simulink model "Vorlage_Gesamtanlage_v27"  (R2021a)
settings: Solver=ode3  StartTime=0.0  StopTime=400  FixedStep=0.01  MaxStep=1  MinStep=0.005  RelTol=1e-3  AbsTol=10  EnableMultiTasking=on
undefined symbols (not defined in the file): A, Flaschengroesse, I, igetr, K, Limits, MaxFlaschen, MRK, numA, PassSilo1, PassSilo2, PHI, Ra, SizeSilo1, SizeSilo2, U, v_band_abfuhr_set, v_band_arbeit_set, v_band_zufuhr_set, v_umsetzer_greifer_set, v_umsetzer_set, v_ve1_set, v_ve2_set
libraries: simulink x94
(part 2 of 3)

== system Vorlage_Gesamtanlage_v27/Abfüllanlage/Fehlererkennung/Leere Flasche durch Ve2 ==
  Leere Flasche durch VE2 : Assertion
  Logical Operator1 : Logic  AllPortsSameDT=off  OutDataTypeStr=boolean
  Logical Operator15 : Logic  Operator=NOT  AllPortsSameDT=off  OutDataTypeStr=boolean
  Memory : Memory  InitialCondition=1  InheritSampleTime=on
  Rising Edge : Subsystem
  nac : Outport
  wires:
  Logical Operator15/1 -> Memory/1
  Memory/1 -> Leere Flasche durch VE2/1
  Logical Operator1/1 -> Logical Operator15/1, nac/1
  Rising Edge/1(edge) -> Logical Operator1/2
  [i_dp_ve2_LT_vorne] -> Logical Operator1/1
  [o_dp_ve2] -> Rising Edge/1(signal)

== system Vorlage_Gesamtanlage_v27/Abfüllanlage/Fehlererkennung/Leere Flasche zurueck ==
  Falling Edge : Subsystem
  Leere Flasche zurueck : Assertion
  Logical Operator12 : Logic  Inputs=3  AllPortsSameDT=off  OutDataTypeStr=boolean
  Logical Operator15 : Logic  Operator=NOT  AllPortsSameDT=off  OutDataTypeStr=boolean
  Memory : Memory  InitialCondition=1  InheritSampleTime=on
  nac : Outport
  wires:
  Memory/1 -> Leere Flasche zurueck/1
  Logical Operator12/1 -> nac/1, Logical Operator15/1
  Logical Operator15/1 -> Memory/1
  Falling Edge/1(edge) -> Logical Operator12/3
  [i_dp_umsetz_teller] -> Falling Edge/1(signal)
  [i_dp_teller_behaelter_vorne] -> Logical Operator12/1
  [i_dp_umsetz_greifer_zu] -> Logical Operator12/2

== system Vorlage_Gesamtanlage_v27/Abfüllanlage/Fehlererkennung/Lückenhafte Teller Bestückung ==
  Compare To Zero : simulink/Logic and Bit Operations/Compare To Zero  relop=>  OutDataTypeStr=boolean
  Interval Test : simulink/Logic and Bit Operations/Interval Test  IntervalClosedRight=off  uplimit=405  IntervalClosedLeft=on  lowlimit=0  OutDataTypeStr=boolean
  Logical Operator : Logic  Operator=NOT  AllPortsSameDT=off  OutDataTypeStr=boolean
  Logical Operator1 : Logic  Inputs=3  AllPortsSameDT=off  OutDataTypeStr=boolean
  Logical Operator2 : Logic  Operator=NOT  AllPortsSameDT=off  OutDataTypeStr=boolean
  Lückehafte Tellerbestückung : Assertion
  Memory2 : Memory  InitialCondition=1  InheritSampleTime=on
  Sum of Elements : Sum  Inputs=+
  rising edge : Subsystem
  nac : Outport
  wires:
  Logical Operator2/1 -> Memory2/1
  Memory2/1 -> Lückehafte Tellerbestückung/1
  [Flaschenpositionen] -> Interval Test/1
  Interval Test/1 -> Sum of Elements/1
  Sum of Elements/1 -> Compare To Zero/1
  [o_dp_teller] -> rising edge/1(In1)
  [i_dp_teller_behaelter_vorne] -> Logical Operator/1
  Logical Operator/1 -> Logical Operator1/1  "keine neue Flasche da"
  rising edge/1(Out1) -> Logical Operator1/2  "teller startet"
  Compare To Zero/1 -> Logical Operator1/3  "neue Flaschen vorhanden"
  Logical Operator1/1 -> nac/1, Logical Operator2/1

== system Vorlage_Gesamtanlage_v27/Abfüllanlage/Fehlererkennung/Nachrieseln ==
  Compare To Constant : simulink/Logic and Bit Operations/Compare To Constant  relop===  const=1  OutDataTypeStr=uint8  ZeroCross=off
  Compare To Constant1 : simulink/Logic and Bit Operations/Compare To Constant  relop=<  const=2  OutDataTypeStr=uint8  ZeroCross=off
  Compare To Constant2 : simulink/Logic and Bit Operations/Compare To Constant  relop=>  const=0  OutDataTypeStr=uint8  ZeroCross=off
  Data Type Conversion : DataTypeConversion
  Integrator : Integrator  ExternalReset=rising
  Logical Operator : Logic  Inputs=3  AllPortsSameDT=off  OutDataTypeStr=boolean
  Logical Operator1 : Logic  Operator=NOT  AllPortsSameDT=off  OutDataTypeStr=boolean
  Logical Operator3 : Logic  Operator=NOT  AllPortsSameDT=off  OutDataTypeStr=boolean
  Memory2 : Memory  InitialCondition=1  InheritSampleTime=on
  Nachrieselzeit missachtet : Assertion
  Rising Edge1 : Subsystem
  nac : Outport
  wires:
  Rising Edge1/1(edge) -> Compare To Constant/1
  Compare To Constant/1 -> Logical Operator/3
  Compare To Constant1/1 -> Logical Operator/2
  Integrator/1 -> Compare To Constant1/1, Compare To Constant2/1
  Logical Operator/1 -> nac/1, Logical Operator3/1
  Logical Operator3/1 -> Memory2/1
  Memory2/1 -> Nachrieselzeit missachtet/1
  [i_dp_BEKenn_LS_oben] -> Logical Operator1/1
  Logical Operator1/1 -> Data Type Conversion/1
  [o_dp_teller] -> Rising Edge1/1(signal)
  Data Type Conversion/1 -> Integrator/1, Integrator/2
  Compare To Constant2/1 -> Logical Operator/1

== system Vorlage_Gesamtanlage_v27/Abfüllanlage/Fehlererkennung/Sinnloser Schaltvorgang Ve1 ==
  CompareTo Constant12 : simulink/Logic and Bit Operations/Compare To Constant  relop===  const=0  OutDataTypeStr=boolean  ZeroCross=off
  Logical Operator1 : Logic  AllPortsSameDT=off  OutDataTypeStr=boolean
  Logical Operator17 : Logic  Operator=NOT  AllPortsSameDT=off  OutDataTypeStr=boolean
  Memory1 : Memory  InitialCondition=1  InheritSampleTime=on
  Rising Edge : Subsystem
  Sinnloser Schaltvorgang VE1 : Assertion
  nac : Outport
  wires:
  [o_dp_ve1] -> Rising Edge/1(signal)
  [i_dp_ve1_LT] -> CompareTo Constant12/1
  Logical Operator1/1 -> nac/1, Logical Operator17/1
  CompareTo Constant12/1 -> Logical Operator1/1
  Rising Edge/1(edge) -> Logical Operator1/2
  Memory1/1 -> Sinnloser Schaltvorgang VE1/1
  Logical Operator17/1 -> Memory1/1

== system Vorlage_Gesamtanlage_v27/Abfüllanlage/Fehlererkennung/Sinnloser Schaltvorgang Ve2 ==
  CompareTo Constant12 : simulink/Logic and Bit Operations/Compare To Constant  relop===  const=0  OutDataTypeStr=boolean  ZeroCross=off
  Logical Operator1 : Logic  AllPortsSameDT=off  OutDataTypeStr=boolean
  Logical Operator17 : Logic  Operator=NOT  AllPortsSameDT=off  OutDataTypeStr=boolean
  Memory1 : Memory  InitialCondition=1  InheritSampleTime=on
  Rising Edge : Subsystem
  Sinnloser Schaltvorgang VE2 : Assertion
  nac2 : Outport
  wires:
  Logical Operator17/1 -> Memory1/1
  Memory1/1 -> Sinnloser Schaltvorgang VE2/1
  Rising Edge/1(edge) -> Logical Operator1/2
  CompareTo Constant12/1 -> Logical Operator1/1
  Logical Operator1/1 -> Logical Operator17/1, nac2/1
  [i_dp_ve2_LT] -> CompareTo Constant12/1
  [o_dp_ve2] -> Rising Edge/1(signal)

== system Vorlage_Gesamtanlage_v27/Abfüllanlage/Fehlererkennung/Teller dreht obwohl Flasche nicht gefuellt ==
  CompareTo Constant11 : simulink/Logic and Bit Operations/Compare To Constant  relop===  const=1  OutDataTypeStr=boolean  ZeroCross=off
  CompareTo Constant12 : simulink/Logic and Bit Operations/Compare To Constant  relop===  const=1  OutDataTypeStr=boolean  ZeroCross=off
  Logical Operator15 : Logic  Operator=NOT  AllPortsSameDT=off  OutDataTypeStr=boolean
  Logical Operator17 : Logic  Inputs=3  AllPortsSameDT=off  OutDataTypeStr=boolean
  Memory : Memory  InitialCondition=1  InheritSampleTime=on
  Rising Edge : Subsystem
  Teller dreht obwohl Flasche nicht gefüllt : Assertion
  nac : Outport
  wires:
  Logical Operator15/1 -> Memory/1
  Memory/1 -> Teller dreht obwohl Flasche nicht gefüllt/1
  CompareTo Constant11/1 -> Logical Operator17/1
  CompareTo Constant12/1 -> Logical Operator17/2
  Rising Edge/1(edge) -> Logical Operator17/3
  Logical Operator17/1 -> Logical Operator15/1, nac/1
  [i_dp_BEKenn_LS_oben] -> CompareTo Constant11/1
  [i_dp_BEKenn_LT_unten] -> CompareTo Constant12/1
  [o_dp_teller] -> Rising Edge/1(signal)

== system Vorlage_Gesamtanlage_v27/Abfüllanlage/Fehlererkennung/Teller dreht obwohl Greifer zu ==
  note: Changelog v23 -> v24:
      | o_dp_umsetz_teller geändert zu i_dp_umsetz_teller
      | o_dp_umsetz_greifer_zu geändert zu i_dp_umsetz_greifer_zu
  Logical Operator14 : Logic  Inputs=4  AllPortsSameDT=off  OutDataTypeStr=boolean
  Logical Operator15 : Logic  Operator=NOT  AllPortsSameDT=off  OutDataTypeStr=boolean
  Memory12 : Memory  InitialCondition=1
  Teller dreht obwohl Greifer zu : Assertion
  nac : Outport
  wires:
  Logical Operator15/1 -> Memory12/1
  Memory12/1 -> Teller dreht obwohl Greifer zu/1
  Logical Operator14/1 -> Logical Operator15/1, nac/1
  [i_dp_umsetz_teller] -> Logical Operator14/1
  [i_dp_umsetz_greifer_zu] -> Logical Operator14/2
  [i_dp_teller_behaelter] -> Logical Operator14/3
  [o_dp_teller] -> Logical Operator14/4

== system Vorlage_Gesamtanlage_v27/Abfüllanlage/Fehlererkennung/Teller dreht volle Flasche durch ==
  Logical Operator1 : Logic  Operator=NOT  AllPortsSameDT=off  OutDataTypeStr=boolean
  Logical Operator2 : Logic  AllPortsSameDT=off  OutDataTypeStr=boolean
  Memory1 : Memory  InitialCondition=1  InheritSampleTime=on
  Rising Edge : Subsystem
  Teller dreht volle Flasche durch : Assertion
  nac1 : Outport
  wires:
  Memory1/1 -> Teller dreht volle Flasche durch/1
  Logical Operator1/1 -> Memory1/1
  Logical Operator2/1 -> Logical Operator1/1, nac1/1
  Rising Edge/1(edge) -> Logical Operator2/2
  [o_dp_teller] -> Rising Edge/1(signal)
  [i_dp_teller_behaelter_hinten] -> Logical Operator2/1

== system Vorlage_Gesamtanlage_v27/Abfüllanlage/Fehlererkennung/Triggered Subsystem13 ==
  Flaschenpositionen : Inport
  CompareTo Constant11 : simulink/Logic and Bit Operations/Compare To Constant  relop=>  const=0  OutDataTypeStr=boolean  ZeroCross=off
  Interval Test10 : simulink/Logic and Bit Operations/Interval Test  IntervalClosedRight=off  uplimit=405.2  IntervalClosedLeft=off  lowlimit=404.8  OutDataTypeStr=boolean
  Sum of Elements9 : Sum  Inputs=+
  i_dp_teller_behaelter_vorne : Outport
  wires:
  Flaschenpositionen/1 -> Interval Test10/1
  Interval Test10/1 -> Sum of Elements9/1
  Sum of Elements9/1 -> CompareTo Constant11/1
  CompareTo Constant11/1 -> i_dp_teller_behaelter_vorne/1

== system Vorlage_Gesamtanlage_v27/Abfüllanlage/Fehlererkennung/Triggered Subsystem14 ==
  Flaschenpositionen : Inport
  CompareTo Constant11 : simulink/Logic and Bit Operations/Compare To Constant  relop=>  const=0  OutDataTypeStr=boolean  ZeroCross=off
  Interval Test10 : simulink/Logic and Bit Operations/Interval Test  IntervalClosedRight=off  uplimit=305.2  IntervalClosedLeft=off  lowlimit=304.8  OutDataTypeStr=boolean
  Sum of Elements9 : Sum  Inputs=+
  i_dp_ve2_LT_vorne : Outport
  wires:
  Flaschenpositionen/1 -> Interval Test10/1
  Interval Test10/1 -> Sum of Elements9/1
  Sum of Elements9/1 -> CompareTo Constant11/1
  CompareTo Constant11/1 -> i_dp_ve2_LT_vorne/1

== system Vorlage_Gesamtanlage_v27/Abfüllanlage/Fehlererkennung/Triggered Subsystem15 ==
  Flaschenpositionen : Inport
  CompareTo Constant11 : simulink/Logic and Bit Operations/Compare To Constant  relop=>  const=0  OutDataTypeStr=boolean  ZeroCross=off
  Interval Test10 : simulink/Logic and Bit Operations/Interval Test  IntervalClosedRight=off  uplimit=505.2  IntervalClosedLeft=off  lowlimit=504.8  OutDataTypeStr=boolean
  Sum of Elements9 : Sum  Inputs=+
  i_dp_teller_behaelter_hinten : Outport
  wires:
  CompareTo Constant11/1 -> i_dp_teller_behaelter_hinten/1
  Sum of Elements9/1 -> CompareTo Constant11/1
  Interval Test10/1 -> Sum of Elements9/1
  Flaschenpositionen/1 -> Interval Test10/1

== system Vorlage_Gesamtanlage_v27/Abfüllanlage/Fehlererkennung/Triggered Subsystem16 ==
  Flaschenpositionen : Inport
  CompareTo Constant11 : simulink/Logic and Bit Operations/Compare To Constant  relop=>  const=0  OutDataTypeStr=boolean  ZeroCross=off
  Interval Test10 : simulink/Logic and Bit Operations/Interval Test  IntervalClosedRight=off  uplimit=605.2  IntervalClosedLeft=off  lowlimit=604.8  OutDataTypeStr=boolean
  Sum of Elements9 : Sum  Inputs=+
  i_dp_ve2_LT_hinten : Outport
  wires:
  Flaschenpositionen/1 -> Interval Test10/1
  Interval Test10/1 -> Sum of Elements9/1
  Sum of Elements9/1 -> CompareTo Constant11/1
  CompareTo Constant11/1 -> i_dp_ve2_LT_hinten/1

== system Vorlage_Gesamtanlage_v27/Abfüllanlage/Fehlererkennung/Umsetzerpneumatik beschädigt ==
  Logical Operator23 : Logic  Operator=NOT  AllPortsSameDT=off  OutDataTypeStr=boolean
  Logical Operator24 : Logic  AllPortsSameDT=off  OutDataTypeStr=boolean
  Memory9 : Memory  InitialCondition=1
  Umsetzerpneumatik beschädigt : Assertion
  nac : Outport
  wires:
  Logical Operator24/1 -> Logical Operator23/1, nac/1
  Logical Operator23/1 -> Memory9/1
  Memory9/1 -> Umsetzerpneumatik beschädigt/1
  [o_dp_umsetz_band] -> Logical Operator24/1
  [o_dp_umsetz_teller] -> Logical Operator24/2

== system Vorlage_Gesamtanlage_v27/Abfüllanlage/Fehlererkennung/Vereinzeler1 schließt mit Flasche ==
  Compare To Constant : simulink/Logic and Bit Operations/Compare To Constant  relop=>=  const=1  OutDataTypeStr=boolean
  Interval Test : simulink/Logic and Bit Operations/Interval Test  IntervalClosedRight=off  uplimit=205  IntervalClosedLeft=off  lowlimit=201  OutDataTypeStr=boolean
  Logical Operator : Logic  AllPortsSameDT=off  OutDataTypeStr=boolean
  Logical Operator2 : Logic  Operator=NOT  AllPortsSameDT=off  OutDataTypeStr=boolean
  Memory2 : Memory  InitialCondition=1  InheritSampleTime=on
  Sum of Elements : Sum  Inputs=+
  Vereinzeler1 schließt mit Flasche : Assertion
  falling edge : Subsystem
  nac : Outport
  wires:
  Memory2/1 -> Vereinzeler1 schließt mit Flasche/1
  Logical Operator2/1 -> Memory2/1
  [o_dp_ve1] -> falling edge/1(In1)
  [Flaschenpositionen] -> Interval Test/1
  Interval Test/1 -> Sum of Elements/1
  Sum of Elements/1 -> Compare To Constant/1
  falling edge/1(Out1) -> Logical Operator/1
  Compare To Constant/1 -> Logical Operator/2
  Logical Operator/1 -> nac/1, Logical Operator2/1

== system Vorlage_Gesamtanlage_v27/Abfüllanlage/Fehlererkennung/Vereinzeler2 schließt mit Flasche1 ==
  Compare To Constant : simulink/Logic and Bit Operations/Compare To Constant  relop=>=  const=1  OutDataTypeStr=boolean
  Interval Test : simulink/Logic and Bit Operations/Interval Test  IntervalClosedRight=off  uplimit=610  IntervalClosedLeft=on  lowlimit=605  OutDataTypeStr=boolean
  Logical Operator : Logic  AllPortsSameDT=off  OutDataTypeStr=boolean
  Logical Operator2 : Logic  Operator=NOT  AllPortsSameDT=off  OutDataTypeStr=boolean
  Memory2 : Memory  InitialCondition=1  InheritSampleTime=on
  Sum of Elements : Sum  Inputs=+
  Vereinzeler2 schließt mit Flasche : Assertion
  falling edge : Subsystem
  nac : Outport
  wires:
  Logical Operator/1 -> nac/1, Logical Operator2/1
  Compare To Constant/1 -> Logical Operator/2
  falling edge/1(Out1) -> Logical Operator/1
  Sum of Elements/1 -> Compare To Constant/1
  Interval Test/1 -> Sum of Elements/1
  [Flaschenpositionen] -> Interval Test/1
  [o_dp_ve2] -> falling edge/1(In1)
  Logical Operator2/1 -> Memory2/1
  Memory2/1 -> Vereinzeler2 schließt mit Flasche/1

== system Vorlage_Gesamtanlage_v27/Abfüllanlage/Fehlererkennung/Volle Flasche zum Teller zurück ==
  Chart : Stateflow chart  TreatAsAtomicUnit=on
  Logical Operator2 : Logic  Operator=NOT  AllPortsSameDT=off  OutDataTypeStr=boolean
  Memory2 : Memory  InitialCondition=1  InheritSampleTime=on
  Scope : Scope
  Volle Flasche zum Teller zurueck : Assertion
  nac : Outport
  wires:
  Logical Operator2/1 -> Memory2/1
  Memory2/1 -> Volle Flasche zum Teller zurueck/1
  Chart/1(error) -> nac/1, Logical Operator2/1
  [i_dp_ve2_herein] -> Scope/1, Chart/6(i_ve2_herein)
  [i_dp_umsetz_band] -> Chart/5(i_umsetz_band)
  [i_dp_umsetz_greifer_auf] -> Chart/4(i_greifer_auf)
  [i_dp_umsetz_teller] -> Chart/3(i_umsetz_teller)
  [i_dp_teller_behaelter_hinten] -> Chart/1(I_teller_behaelter_hinten)
  [i_dp_umsetz_greifer_zu] -> Chart/2(i_greifer_zu)
  [o_dp_umsetz_teller] -> Chart/7(o_umsetz_teller)

== system Vorlage_Gesamtanlage_v27/Abfüllanlage/Fehlererkennung/Volle Flasche zurueck ==
  Falling Edge : Subsystem
  Logical Operator1 : Logic  Inputs=3  AllPortsSameDT=off  OutDataTypeStr=boolean
  Logical Operator15 : Logic  Operator=NOT  AllPortsSameDT=off  OutDataTypeStr=boolean
  Memory : Memory  InitialCondition=1  InheritSampleTime=on
  Volle Flasche zurueck : Assertion
  nac : Outport
  wires:
  Logical Operator15/1 -> Memory/1
  Logical Operator1/1 -> Logical Operator15/1, nac/1
  Memory/1 -> Volle Flasche zurueck/1
  Falling Edge/1(edge) -> Logical Operator1/3
  [i_dp_umsetz_band] -> Falling Edge/1(signal)
  [i_dp_ve2_LT_hinten] -> Logical Operator1/1
  [i_dp_umsetz_greifer_zu] -> Logical Operator1/2

== system Vorlage_Gesamtanlage_v27/Abfüllanlage/Fehlererkennung/Zwei Flaschen im Umsetzer1 ==
  CompareTo Constant2 : simulink/Logic and Bit Operations/Compare To Constant  relop=>  const=1  OutDataTypeStr=boolean  ZeroCross=off
  Interval Test2 : simulink/Logic and Bit Operations/Interval Test  IntervalClosedRight=off  uplimit=405  IntervalClosedLeft=on  lowlimit=306  OutDataTypeStr=boolean
  Logical Operator2 : Logic  Operator=NOT  AllPortsSameDT=off  OutDataTypeStr=boolean
  Memory4 : Memory  InitialCondition=1
  Sum of Elements2 : Sum  Inputs=+
  Zwei Flaschen im Umsetzer1 : Assertion
  nac : Outport
  wires:
  Sum of Elements2/1 -> CompareTo Constant2/1
  Interval Test2/1 -> Sum of Elements2/1
  Logical Operator2/1 -> Memory4/1
  CompareTo Constant2/1 -> Logical Operator2/1, nac/1
  Memory4/1 -> Zwei Flaschen im Umsetzer1/1
  [Flaschenpositionen] -> Interval Test2/1

== system Vorlage_Gesamtanlage_v27/Abfüllanlage/Fehlererkennung/Zwei Flaschen im Umsetzer2 ==
  CompareTo Constant3 : simulink/Logic and Bit Operations/Compare To Constant  relop=>  const=1  OutDataTypeStr=boolean  ZeroCross=off
  Interval Test3 : simulink/Logic and Bit Operations/Interval Test  IntervalClosedRight=off  uplimit=604  IntervalClosedLeft=on  lowlimit=505  OutDataTypeStr=boolean
  Logical Operator3 : Logic  Operator=NOT  AllPortsSameDT=off  OutDataTypeStr=boolean
  Memory3 : Memory  InitialCondition=1
  Sum of Elements3 : Sum  Inputs=+
  Zwei Flaschen im Umsetzer2 : Assertion
  nac : Outport
  wires:
  Sum of Elements3/1 -> CompareTo Constant3/1
  Interval Test3/1 -> Sum of Elements3/1
  Logical Operator3/1 -> Memory3/1
  CompareTo Constant3/1 -> Logical Operator3/1, nac/1
  Memory3/1 -> Zwei Flaschen im Umsetzer2/1
  [Flaschenpositionen] -> Interval Test3/1

== system Vorlage_Gesamtanlage_v27/Abfüllanlage/Fehlererkennung/Zwei Flaschen im Ve1 ==
  CompareTo Constant : simulink/Logic and Bit Operations/Compare To Constant  relop=>  const=1  OutDataTypeStr=boolean  ZeroCross=off
  Interval Test : simulink/Logic and Bit Operations/Interval Test  IntervalClosedRight=off  uplimit=205  IntervalClosedLeft=on  lowlimit=201  OutDataTypeStr=boolean
  Logical Operator : Logic  Operator=NOT  AllPortsSameDT=off  OutDataTypeStr=boolean
  Memory6 : Memory  InitialCondition=1
  Sum of Elements : Sum  Inputs=+
  Zwei Flaschen im Ve1 : Assertion
  nac : Outport
  wires:
  Memory6/1 -> Zwei Flaschen im Ve1/1
  CompareTo Constant/1 -> Logical Operator/1, nac/1
  Logical Operator/1 -> Memory6/1
  Interval Test/1 -> Sum of Elements/1
  Sum of Elements/1 -> CompareTo Constant/1
  [Flaschenpositionen] -> Interval Test/1

== system Vorlage_Gesamtanlage_v27/Abfüllanlage/Fehlererkennung/Zwei Flaschen im Ve2 ==
  CompareTo Constant1 : simulink/Logic and Bit Operations/Compare To Constant  relop=>  const=1  OutDataTypeStr=boolean  ZeroCross=off
  Interval Test1 : simulink/Logic and Bit Operations/Interval Test  IntervalClosedRight=off  uplimit=610  IntervalClosedLeft=on  lowlimit=605  OutDataTypeStr=boolean
  Interval Test2 : simulink/Logic and Bit Operations/Interval Test  IntervalClosedRight=off  uplimit=305  IntervalClosedLeft=on  lowlimit=300  OutDataTypeStr=boolean
  Logical Operator : Logic  Operator=OR  AllPortsSameDT=off  OutDataTypeStr=boolean
  Logical Operator1 : Logic  Operator=NOT  AllPortsSameDT=off  OutDataTypeStr=boolean
  Memory5 : Memory  InitialCondition=1
  Sum of Elements1 : Sum  Inputs=+
  Zwei Flaschen im Ve2 : Assertion
  nac : Outport
  wires:
  Sum of Elements1/1 -> CompareTo Constant1/1
  Logical Operator1/1 -> Memory5/1
  CompareTo Constant1/1 -> Logical Operator1/1, nac/1
  Memory5/1 -> Zwei Flaschen im Ve2/1
  [Flaschenpositionen] -> Interval Test1/1, Interval Test2/1
  Interval Test1/1 -> Logical Operator/1
  Interval Test2/1 -> Logical Operator/2
  Logical Operator/1 -> Sum of Elements1/1

== system Vorlage_Gesamtanlage_v27/Abfüllanlage/Fehlererkennung/nac ==
  nac : Inport
  Constant : Constant  Value=numA
  Data Type Conversion2 : DataTypeConversion  OutDataTypeStr=double
  Display : Display
  Increment Stored Integer : simulink/Additional Math & Discrete/Additional Math: Increment - Decrement/Increment Stored Integer
  MinMax : MinMax  Function=max  Inputs=2
  Product1 : Product  RndMeth=Zero
  To Workspace : ToWorkspace  VariableName=numA  SampleTime=-1
      settings: MaxDataPoints=1
  wires:
  nac/1 -> Data Type Conversion2/1
  MinMax/1 -> Display/1, To Workspace/1
  Constant/1 -> Increment Stored Integer/1, MinMax/1
  Increment Stored Integer/1 -> Product1/1
  Data Type Conversion2/1 -> Product1/2
  Product1/1 -> MinMax/2

== system Vorlage_Gesamtanlage_v27/Abfüllanlage/Flaschen_data/Flaschengeschwindigkeiten ==
  Anlagengeschwindigkeiten : Inport
  i_dp_umsetz_greifer_zu : Inport  Port=2
  Flaschenpositionen : Inport  Port=3
  umsetz_pos : Inport  Port=4
  Anlagenpositionsbestimmung : Subsystem
  Filter : Subsystem
  Flaschenabstandsüberwachung : Subsystem
  Product : Product  RndMeth=Zero  SaturateOnIntegerOverflow=on  OutDataTypeStr=Inherit: Same as first input
  Selector : Selector  InputPortWidth=10  IndexOptions=Index vector (port)  Indices=[1 3]  OutputSizes=1
  Flaschengeschwindigkeiten : Outport
  Anlagenpositionen : Outport  Port=2
  tag scope: Anlagenposition=global, Flaschenanlagengeschwindigkeiten=global
  wires:
  Flaschenpositionen/1 -> Anlagenpositionsbestimmung/1(Flaschenposition), Flaschenabstandsüberwachung/1(Flaschenpostionen)
  Anlagenpositionsbestimmung/1(Anlagenposition) -> Selector/2, [Anlagenposition], Anlagenpositionen/1
  Anlagengeschwindigkeiten/1 -> Filter/1(Anlagengeschwindigkeiten)
  Filter/1(Flaschenanlagengeschwindigkeiten) -> Selector/1, [Flaschenanlagengeschwindigkeiten]
  i_dp_umsetz_greifer_zu/1 -> Filter/2(i_dp_umsetz_greifer_zu)
  Flaschenabstandsüberwachung/1(Bewegung möglich) -> Product/2
  Selector/1 -> Product/1
  Product/1 -> Flaschengeschwindigkeiten/1
  umsetz_pos/1 -> Flaschenabstandsüberwachung/2(umsetz_pos)

== system Vorlage_Gesamtanlage_v27/Abfüllanlage/Flaschen_data/Flaschenstarter ==
  Flaschenpositionen : Inport
  Flasche : Inport  Port=2
  Constant : Constant  OutDataTypeStr=uint16
  Flaschenstarter : Subsystem
  Math Function : Math  Operator=mod  SignedPower=on  SaturateOnIntegerOverflow=on
  Maximale Flaschenanzahl : Constant  Value=MaxFlaschen  OutDataTypeStr=uint16
  Memory : Memory  InitialCondition=1
  Sum1 : Sum  Inputs=|++  SaturateOnIntegerOverflow=on
  in_Flaschenzähler : Subsystem
  Flaschenpositionen mit Starter : Outport
  tag scope: Flaschenanzahl=global
  wires:
  in_Flaschenzähler/2(Count) -> Math Function/1
  Maximale Flaschenanzahl/1 -> Math Function/2
  Math Function/1 -> [Flaschenanzahl], Sum1/1
  in_Flaschenzähler/1(Rising Edge) -> Flaschenstarter/3(Rising_edge von Flasche)
  Sum1/1 -> Memory/1
  Constant/1 -> Sum1/2
  Memory/1 -> Flaschenstarter/2(Flaschenanzahl)
  Flaschenpositionen/1 -> Flaschenstarter/1(Flaschenpositionen)
  Flaschenstarter/1(Flaschenpositionen mit Starter) -> Flaschenpositionen mit Starter/1
  Flasche/1 -> in_Flaschenzähler/1(Signal)

== system Vorlage_Gesamtanlage_v27/Abfüllanlage/Flaschen_data/v -> x ==
  Flaschengeschwindigkeiten : Inport
  Anlagenpositionen : Inport  Port=2
  Anlagenlimits : Inport  Port=3
  Compare To Zero : simulink/Logic and Bit Operations/Compare To Zero  relop=>  OutDataTypeStr=boolean  ZeroCross=off
  Data Type Conversion : DataTypeConversion
  Derivative : Derivative
  Gain : Gain  Gain=0
  Integrator : Integrator  ExternalReset=rising  InitialConditionSource=external  InitialCondition=zeros(25,1)  UpperSaturationLimit=Limits  LowerSaturationLimit=[0 0 0]
  Memory : Memory  InitialCondition=ones(25,1)*100
  Memory1 : Memory  InitialCondition=ones(25,1)
  Saturation Dynamic : simulink/Discontinuities/Saturation Dynamic  OutMin=[]  OutMax=[]  OutDataTypeStr=Inherit: Same as second input  OutDataType=sfix(16)  OutScaling=2^-10  DoSatur=off
  Selector : Selector  InputPortWidth=10  IndexOptions=Index vector (port)  Indices=[1 3]  OutputSizes=1
  Flaschenpositionen : Outport
  wires:
  Flaschengeschwindigkeiten/1 -> Integrator/1
  Gain/1 -> Saturation Dynamic/3
  Derivative/1 -> Compare To Zero/1
  Compare To Zero/1 -> Data Type Conversion/1
  Anlagenlimits/1 -> Selector/1
  Integrator/1 -> Saturation Dynamic/2
  Saturation Dynamic/1 -> Flaschenpositionen/1
  Anlagenpositionen/1 -> Memory1/1
  Selector/1 -> Derivative/1, Gain/1, Saturation Dynamic/1, Memory/1
  Memory1/1 -> Selector/2
  Memory/1 -> Integrator/3
  Data Type Conversion/1 -> Integrator/2

== system Vorlage_Gesamtanlage_v27/Abfüllanlage/Umsetzgreifer/Greifer ==
  o_dp_umsetz_greifer_auf : Inport
  o_dp_umsetz_greifer_zu : Inport  Port=2
  Compare To Constant2 : simulink/Logic and Bit Operations/Compare To Constant  relop=>=  const=100  OutDataTypeStr=boolean  ZeroCross=off
  Compare To Constant3 : simulink/Logic and Bit Operations/Compare To Constant  relop=<=  const=0  OutDataTypeStr=boolean  ZeroCross=off
  Derivative : Derivative
  Gain2 : Gain  Gain=v_umsetzer_greifer_set
  Integrator1 : Integrator  LimitOutput=on  UpperSaturationLimit=100  LowerSaturationLimit=0
  Subtract1 : Sum  Inputs=+-
  i_dp_umsetz_greifer_auf : Outport  OutDataTypeStr=boolean
  i_dp_umsetz_greifer_zu : Outport  Port=2  OutDataTypeStr=boolean
  tag scope: i_dp_umsetz_greifer_auf=global, i_dp_umsetz_greifer_zu=global, o_dp_umsetz_greifer_auf=global, o_dp_umsetz_greifer_zu=global, s_Greifer=global, v_Greifer=global
  wires:
  Gain2/1 -> Integrator1/1
  Subtract1/1 -> Gain2/1
  Integrator1/1 -> Compare To Constant3/1, [s_Greifer], Compare To Constant2/1, Derivative/1
  o_dp_umsetz_greifer_zu/1 -> Subtract1/2, [o_dp_umsetz_greifer_zu]
  o_dp_umsetz_greifer_auf/1 -> Subtract1/1, [o_dp_umsetz_greifer_auf]
  Compare To Constant2/1 -> i_dp_umsetz_greifer_auf/1, [i_dp_umsetz_greifer_auf]
  Compare To Constant3/1 -> i_dp_umsetz_greifer_zu/1, [i_dp_umsetz_greifer_zu]
  Derivative/1 -> [v_Greifer]

== system Vorlage_Gesamtanlage_v27/Abfüllanlage/Umsetzgreifer/Umsetzer ==
  o_dp_umsetz_band : Inport
  o_dp_umsetz_teller : Inport  Port=2
  Compare To Constant : simulink/Logic and Bit Operations/Compare To Constant  relop=>=  const=100  OutDataTypeStr=boolean  ZeroCross=off
  Compare To Constant1 : simulink/Logic and Bit Operations/Compare To Constant  relop=<=  const=0  OutDataTypeStr=boolean  ZeroCross=off
  Derivative : Derivative
  Gain : Gain  Gain=-v_umsetzer_set
  Integrator : Integrator  InitialCondition=100  LimitOutput=on  UpperSaturationLimit=101  LowerSaturationLimit=0
  Subtract : Sum  Inputs=+-
  v_umsetzer : Outport  OutDataTypeStr=double
  i_dp_umsetz_teller : Outport  Port=2  OutDataTypeStr=boolean
  i_dp_umsetz_band : Outport  Port=3  OutDataTypeStr=boolean
  umsetz_pos : Outport  Port=4  OutDataTypeStr=double
  tag scope: i_dp_umsetz_band=global, i_dp_umsetz_teller=global, o_dp_umsetz_band=global, o_dp_umsetz_teller=global, s_umsetzer=global, v_umsetzer=global
  wires:
  Gain/1 -> Integrator/1
  Subtract/1 -> Gain/1
  Integrator/1 -> Compare To Constant/1, Derivative/1, Compare To Constant1/1, [s_umsetzer], umsetz_pos/1
  o_dp_umsetz_band/1 -> Subtract/1, [o_dp_umsetz_band]
  o_dp_umsetz_teller/1 -> Subtract/2, [o_dp_umsetz_teller]
  Derivative/1 -> v_umsetzer/1, [v_umsetzer]
  Compare To Constant/1 -> i_dp_umsetz_teller/1, [i_dp_umsetz_teller]
  Compare To Constant1/1 -> i_dp_umsetz_band/1, [i_dp_umsetz_band]

== system Vorlage_Gesamtanlage_v27/Auswertung/Gesamt/Flaschenpositionen ==
  Flaschenpositionen : Scope
  To Workspace : ToWorkspace  VariableName=Flaschenpositionen  SaveFormat=Structure With Time  SampleTime=-1
  wires:
  [Flaschenpositionen] -> Flaschenpositionen/1, To Workspace/1  "Flaschenpositionen"

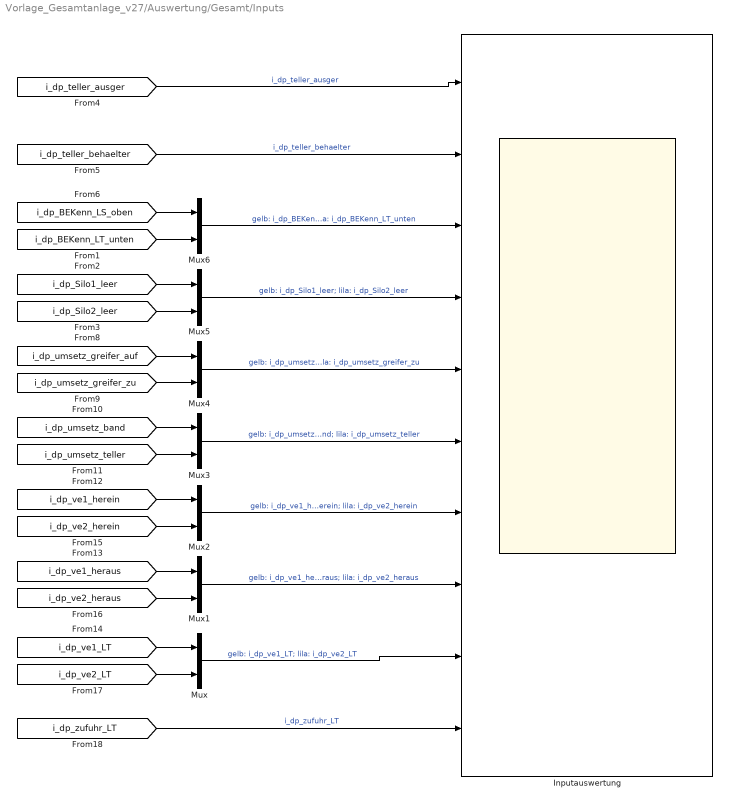
== system Vorlage_Gesamtanlage_v27/Auswertung/Gesamt/Inputs ==
  Inputauswertung : Scope  NumInputPorts=10
  Mux{,1..6} (7 alike) : Mux  Inputs=2
  wires:
  [i_dp_ve1_LT] -> Mux/1
  [i_dp_ve2_LT] -> Mux/2
  [i_dp_ve1_heraus] -> Mux1/1
  [i_dp_ve2_heraus] -> Mux1/2
  [i_dp_ve1_herein] -> Mux2/1
  [i_dp_ve2_herein] -> Mux2/2
  [i_dp_umsetz_band] -> Mux3/1
  [i_dp_umsetz_teller] -> Mux3/2
  [i_dp_umsetz_greifer_auf] -> Mux4/1
  [i_dp_umsetz_greifer_zu] -> Mux4/2
  [i_dp_Silo1_leer] -> Mux5/1
  [i_dp_Silo2_leer] -> Mux5/2
  [i_dp_BEKenn_LS_oben] -> Mux6/1
  [i_dp_BEKenn_LT_unten] -> Mux6/2
  [i_dp_teller_ausger] -> Inputauswertung/1  "i_dp_teller_ausger"
  [i_dp_teller_behaelter] -> Inputauswertung/2  "i_dp_teller_behaelter"
  Mux6/1 -> Inputauswertung/3  "gelb: i_dp_BEKenn_LS_oben; lila: i_dp_BEKenn_LT_unten"
  Mux5/1 -> Inputauswertung/4  "gelb: i_dp_Silo1_leer; lila: i_dp_Silo2_leer"
  Mux4/1 -> Inputauswertung/5  "gelb: i_dp_umsetz_greifer_auf; lila: i_dp_umsetz_greifer_zu"
  Mux3/1 -> Inputauswertung/6  "gelb: i_dp_umsetz_band; lila: i_dp_umsetz_teller"
  Mux2/1 -> Inputauswertung/7  "gelb: i_dp_ve1_herein; lila: i_dp_ve2_herein"
  Mux1/1 -> Inputauswertung/8  "gelb: i_dp_ve1_heraus; lila: i_dp_ve2_heraus"
  [i_dp_zufuhr_LT] -> Inputauswertung/10  "i_dp_zufuhr_LT"
  Mux/1 -> Inputauswertung/9  "gelb: i_dp_ve1_LT; lila: i_dp_ve2_LT"

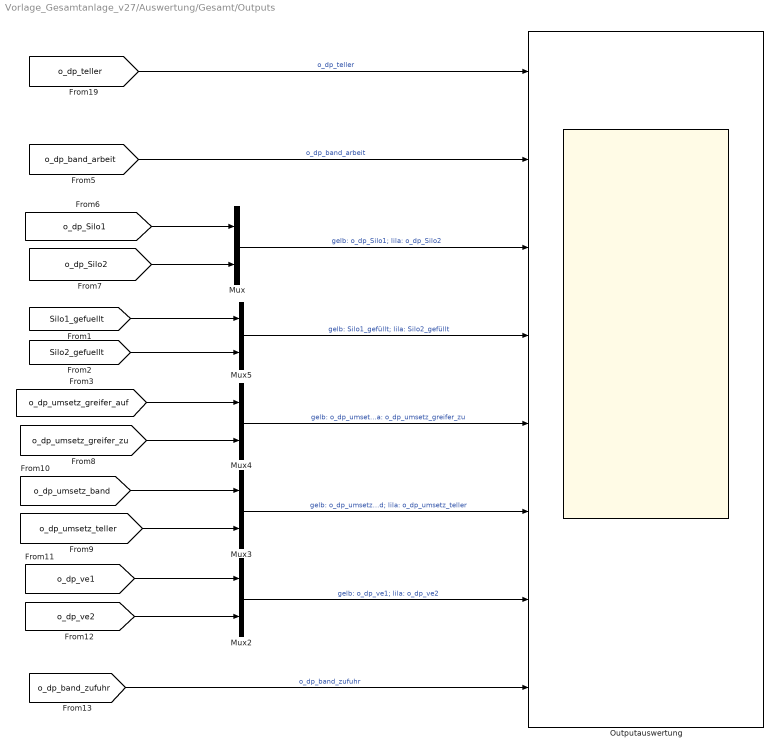
== system Vorlage_Gesamtanlage_v27/Auswertung/Gesamt/Outputs ==
  Mux{,2..5} (5 alike) : Mux  Inputs=2
  Outputauswertung : Scope  NumInputPorts=8
  wires:
  Mux2/1 -> Outputauswertung/7  "gelb: o_dp_ve1; lila: o_dp_ve2"
  Mux3/1 -> Outputauswertung/6  "gelb: o_dp_umsetz_band; lila: o_dp_umsetz_teller"
  Mux4/1 -> Outputauswertung/5  "gelb: o_dp_umsetz_greifer_auf; lila: o_dp_umsetz_greifer_zu"
  Mux5/1 -> Outputauswertung/4  "gelb: Silo1_gefüllt; lila: Silo2_gefüllt"
  [o_dp_band_arbeit] -> Outputauswertung/2  "o_dp_band_arbeit"
  [o_dp_teller] -> Outputauswertung/1  "o_dp_teller"
  [o_dp_umsetz_greifer_zu] -> Mux4/2
  [o_dp_umsetz_greifer_auf] -> Mux4/1
  [o_dp_umsetz_band] -> Mux3/1
  [o_dp_umsetz_teller] -> Mux3/2
  [Silo2_gefuellt] -> Mux5/2
  [Silo1_gefuellt] -> Mux5/1
  [o_dp_ve1] -> Mux2/1
  [o_dp_ve2] -> Mux2/2
  Mux/1 -> Outputauswertung/3  "gelb: o_dp_Silo1; lila: o_dp_Silo2"
  [o_dp_Silo2] -> Mux/2
  [o_dp_Silo1] -> Mux/1
  [o_dp_band_zufuhr] -> Outputauswertung/8  "o_dp_band_zufuhr"

== system Vorlage_Gesamtanlage_v27/Auswertung/Silo/Gesamt ==
  Gesamtsiloauswertung : Scope  NumInputPorts=3
  wires:
  [Fuellmenge_Flasche] -> Gesamtsiloauswertung/1  "eingefüllte Menge in Flasche"
  [i_dp_BEKenn_LS_oben] -> Gesamtsiloauswertung/2  "i_dp_BEKenn_LS_oben"
  [i_dp_BEKenn_LT_unten] -> Gesamtsiloauswertung/3  "i_dp_BEKenn_LT_unten"

== system Vorlage_Gesamtanlage_v27/Auswertung/Silo/Silo1 ==
  Auswertung von Silo 1 : Scope  NumInputPorts=5
  wires:
  [Durchlauf_Silo1] -> Auswertung von Silo 1/1  "Durchlauf Silo 1"
  [o_dp_Silo1] -> Auswertung von Silo 1/2  "o_dp_Silo1"
  [Silo1_gefuellt] -> Auswertung von Silo 1/3  "Silo 1 gefüllt"
  [Fehlmenge_Silo1] -> Auswertung von Silo 1/4  "Fehlmenge Silo 1"
  [i_dp_Silo1_leer] -> Auswertung von Silo 1/5  "i_dp_Silo1_leer"

== system Vorlage_Gesamtanlage_v27/Auswertung/Silo/Silo2 ==
  Auswertung von Silo 2 : Scope  NumInputPorts=5
  wires:
  [i_dp_Silo2_leer] -> Auswertung von Silo 2/5  "i_dp_Silo2_leer"
  [Fehlmenge_Silo2] -> Auswertung von Silo 2/4  "Fehlmenge Silo 2"
  [Silo2_gefuellt] -> Auswertung von Silo 2/3  "Silo 2 gefüllt"
  [o_dp_Silo2] -> Auswertung von Silo 2/2  "o_dp_Silo2"
  [Durchlauf_Silo2] -> Auswertung von Silo 2/1  "Durchlauf Silo 2"

== system Vorlage_Gesamtanlage_v27/Auswertung/Umsetzgreifer/Gesamt ==
  Umsetzgreiferauswertung : Scope  NumInputPorts=5
  wires:
  [v_umsetzer] -> Umsetzgreiferauswertung/1  "Umsetzergeschwindigkeit"
  [s_umsetzer] -> Umsetzgreiferauswertung/2  "Umsetzerweg"
  [v_Greifer] -> Umsetzgreiferauswertung/3  "Greifergeschwindigkeit"
  [s_Greifer] -> Umsetzgreiferauswertung/4  "Greiferweg"
  [i_dp_umsetz_greifer_zu] -> Umsetzgreiferauswertung/5  "i_dp_umsetz_greifer_zu"

== system Vorlage_Gesamtanlage_v27/Auswertung/Umsetzgreifer/Greifer ==
  Greiferauswertung : Scope  NumInputPorts=6
  wires:
  [v_Greifer] -> Greiferauswertung/1  "Greifergeschwindigkeit"
  [s_Greifer] -> Greiferauswertung/2  "Greiferweg"
  [o_dp_umsetz_greifer_auf] -> Greiferauswertung/3  "o_dp_umsetz_greifer_auf"
  [o_dp_umsetz_greifer_zu] -> Greiferauswertung/4  "o_dp_umsetz_greifer_zu"
  [i_dp_umsetz_greifer_auf] -> Greiferauswertung/5  "i_dp_umsetz_greifer_auf"
  [i_dp_umsetz_greifer_zu] -> Greiferauswertung/6  "i_dp_umsetz_greifer_zu"

== system Vorlage_Gesamtanlage_v27/Auswertung/Umsetzgreifer/Umsetzer ==
  Umsetzerauswertung : Scope  NumInputPorts=6
  wires:
  [i_dp_umsetz_band] -> Umsetzerauswertung/5  "i_dp_umsetz_band"
  [o_dp_umsetz_teller] -> Umsetzerauswertung/4  "o_dp_umsetz_teller"
  [o_dp_umsetz_band] -> Umsetzerauswertung/3  "o_dp_umsetz_band"
  [s_umsetzer] -> Umsetzerauswertung/2  "Umsetzerweg"
  [v_umsetzer] -> Umsetzerauswertung/1  "Umsetzergeschwindigkeit"
  [i_dp_umsetz_teller] -> Umsetzerauswertung/6  "i_dp_umsetz_teller"

== system Vorlage_Gesamtanlage_v27/Abfüllanlage/Fehlererkennung/Flasche am Band umgeworfen/Rising Edge ==
  signal : Inport
  Logical Operator : Logic  AllPortsSameDT=off  OutDataTypeStr=boolean
  Logical Operator1 : Logic  Operator=NOT  AllPortsSameDT=off  OutDataTypeStr=boolean
  Memory : Memory
  edge : Outport
  wires:
  Memory/1 -> Logical Operator1/1
  Logical Operator1/1 -> Logical Operator/2
  signal/1 -> Memory/1, Logical Operator/1
  Logical Operator/1 -> edge/1

== system Vorlage_Gesamtanlage_v27/Abfüllanlage/Fehlererkennung/Flasche am Teller umgeworfen/Rising Edge ==
  signal : Inport
  Logical Operator : Logic  AllPortsSameDT=off  OutDataTypeStr=boolean
  Logical Operator1 : Logic  Operator=NOT  AllPortsSameDT=off  OutDataTypeStr=boolean
  Memory : Memory
  edge : Outport
  wires:
  Memory/1 -> Logical Operator1/1
  Logical Operator1/1 -> Logical Operator/2
  signal/1 -> Memory/1, Logical Operator/1
  Logical Operator/1 -> edge/1

== system Vorlage_Gesamtanlage_v27/Abfüllanlage/Fehlererkennung/Flasche trifft Greifer am Band/Rising Edge ==
  signal : Inport
  Logical Operator : Logic  AllPortsSameDT=off  OutDataTypeStr=boolean
  Logical Operator1 : Logic  Operator=NOT  AllPortsSameDT=off  OutDataTypeStr=boolean
  Memory : Memory
  edge : Outport
  wires:
  Memory/1 -> Logical Operator1/1
  Logical Operator1/1 -> Logical Operator/2
  signal/1 -> Memory/1, Logical Operator/1
  Logical Operator/1 -> edge/1

== system Vorlage_Gesamtanlage_v27/Abfüllanlage/Fehlererkennung/Flasche trifft Greifer am Teller/Rising Edge ==
  signal : Inport
  Logical Operator : Logic  AllPortsSameDT=off  OutDataTypeStr=boolean
  Logical Operator1 : Logic  Operator=NOT  AllPortsSameDT=off  OutDataTypeStr=boolean
  Memory : Memory
  edge : Outport
  wires:
  Memory/1 -> Logical Operator1/1
  Logical Operator1/1 -> Logical Operator/2
  signal/1 -> Memory/1, Logical Operator/1
  Logical Operator/1 -> edge/1

== system Vorlage_Gesamtanlage_v27/Abfüllanlage/Fehlererkennung/Greifer geschlossen ohne Flasche/Rising Edge ==
  signal : Inport
  Logical Operator : Logic  AllPortsSameDT=off  OutDataTypeStr=boolean
  Logical Operator1 : Logic  Operator=NOT  AllPortsSameDT=off  OutDataTypeStr=boolean
  Memory : Memory
  edge : Outport
  wires:
  Logical Operator/1 -> edge/1
  signal/1 -> Logical Operator/1, Memory/1
  Logical Operator1/1 -> Logical Operator/2
  Memory/1 -> Logical Operator1/1

== system Vorlage_Gesamtanlage_v27/Abfüllanlage/Fehlererkennung/Leere Flasche durch Ve2/Rising Edge ==
  signal : Inport
  Logical Operator : Logic  AllPortsSameDT=off  OutDataTypeStr=boolean
  Logical Operator1 : Logic  Operator=NOT  AllPortsSameDT=off  OutDataTypeStr=boolean
  Memory : Memory
  edge : Outport
  wires:
  Memory/1 -> Logical Operator1/1
  Logical Operator1/1 -> Logical Operator/2
  signal/1 -> Memory/1, Logical Operator/1
  Logical Operator/1 -> edge/1

== system Vorlage_Gesamtanlage_v27/Abfüllanlage/Fehlererkennung/Leere Flasche zurueck/Falling Edge ==
  signal : Inport
  Logical Operator : Logic  AllPortsSameDT=off  OutDataTypeStr=boolean
  Logical Operator2 : Logic  Operator=NOT  AllPortsSameDT=off  OutDataTypeStr=boolean
  Memory : Memory
  edge : Outport
  wires:
  Logical Operator/1 -> edge/1
  signal/1 -> Memory/1, Logical Operator2/1
  Memory/1 -> Logical Operator/2
  Logical Operator2/1 -> Logical Operator/1

== system Vorlage_Gesamtanlage_v27/Abfüllanlage/Fehlererkennung/Lückenhafte Teller Bestückung/rising edge ==
  In1 : Inport
  Logical Operator : Logic  AllPortsSameDT=off  OutDataTypeStr=boolean
  Logical Operator1 : Logic  Operator=NOT  AllPortsSameDT=off  OutDataTypeStr=boolean
  Memory : Memory
  Out1 : Outport
  wires:
  In1/1 -> Logical Operator/2, Logical Operator1/1
  Memory/1 -> Logical Operator/1
  Logical Operator1/1 -> Memory/1
  Logical Operator/1 -> Out1/1

== system Vorlage_Gesamtanlage_v27/Abfüllanlage/Fehlererkennung/Nachrieseln/Rising Edge1 ==
  signal : Inport
  Logical Operator : Logic  AllPortsSameDT=off  OutDataTypeStr=boolean
  Logical Operator1 : Logic  Operator=NOT  AllPortsSameDT=off  OutDataTypeStr=boolean
  Memory : Memory
  edge : Outport
  wires:
  Memory/1 -> Logical Operator1/1
  Logical Operator1/1 -> Logical Operator/2
  signal/1 -> Memory/1, Logical Operator/1
  Logical Operator/1 -> edge/1

== system Vorlage_Gesamtanlage_v27/Abfüllanlage/Fehlererkennung/Sinnloser Schaltvorgang Ve1/Rising Edge ==
  signal : Inport
  Logical Operator : Logic  AllPortsSameDT=off  OutDataTypeStr=boolean
  Logical Operator1 : Logic  Operator=NOT  AllPortsSameDT=off  OutDataTypeStr=boolean
  Memory : Memory
  edge : Outport
  wires:
  Logical Operator/1 -> edge/1
  signal/1 -> Logical Operator/1, Memory/1
  Logical Operator1/1 -> Logical Operator/2
  Memory/1 -> Logical Operator1/1

== system Vorlage_Gesamtanlage_v27/Abfüllanlage/Fehlererkennung/Sinnloser Schaltvorgang Ve2/Rising Edge ==
  signal : Inport
  Logical Operator : Logic  AllPortsSameDT=off  OutDataTypeStr=boolean
  Logical Operator1 : Logic  Operator=NOT  AllPortsSameDT=off  OutDataTypeStr=boolean
  Memory : Memory
  edge : Outport
  wires:
  Memory/1 -> Logical Operator1/1
  Logical Operator1/1 -> Logical Operator/2
  signal/1 -> Memory/1, Logical Operator/1
  Logical Operator/1 -> edge/1

== system Vorlage_Gesamtanlage_v27/Abfüllanlage/Fehlererkennung/Teller dreht obwohl Flasche nicht gefuellt/Rising Edge ==
  signal : Inport
  Logical Operator : Logic  AllPortsSameDT=off  OutDataTypeStr=boolean
  Logical Operator1 : Logic  Operator=NOT  AllPortsSameDT=off  OutDataTypeStr=boolean
  Memory : Memory
  edge : Outport
  wires:
  Memory/1 -> Logical Operator1/1
  Logical Operator1/1 -> Logical Operator/2
  signal/1 -> Memory/1, Logical Operator/1
  Logical Operator/1 -> edge/1

== system Vorlage_Gesamtanlage_v27/Abfüllanlage/Fehlererkennung/Teller dreht volle Flasche durch/Rising Edge ==
  signal : Inport
  Logical Operator : Logic  AllPortsSameDT=off  OutDataTypeStr=boolean
  Logical Operator1 : Logic  Operator=NOT  AllPortsSameDT=off  OutDataTypeStr=boolean
  Memory : Memory
  edge : Outport
  wires:
  Logical Operator/1 -> edge/1
  signal/1 -> Logical Operator/1, Memory/1
  Logical Operator1/1 -> Logical Operator/2
  Memory/1 -> Logical Operator1/1

== system Vorlage_Gesamtanlage_v27/Abfüllanlage/Fehlererkennung/Vereinzeler1 schließt mit Flasche/falling edge ==
  In1 : Inport
  Logical Operator : Logic  AllPortsSameDT=off  OutDataTypeStr=boolean
  Logical Operator1 : Logic  Operator=NOT  AllPortsSameDT=off  OutDataTypeStr=boolean
  Memory : Memory
  Out1 : Outport
  wires:
  In1/1 -> Memory/1, Logical Operator1/1
  Memory/1 -> Logical Operator/2
  Logical Operator1/1 -> Logical Operator/1
  Logical Operator/1 -> Out1/1

== system Vorlage_Gesamtanlage_v27/Abfüllanlage/Fehlererkennung/Vereinzeler2 schließt mit Flasche1/falling edge ==
  In1 : Inport
  Logical Operator : Logic  AllPortsSameDT=off  OutDataTypeStr=boolean
  Logical Operator1 : Logic  Operator=NOT  AllPortsSameDT=off  OutDataTypeStr=boolean
  Memory : Memory
  Out1 : Outport
  wires:
  Logical Operator/1 -> Out1/1
  Logical Operator1/1 -> Logical Operator/1
  Memory/1 -> Logical Operator/2
  In1/1 -> Logical Operator1/1, Memory/1

== system Vorlage_Gesamtanlage_v27/Abfüllanlage/Fehlererkennung/Volle Flasche zurueck/Falling Edge ==
  signal : Inport
  Logical Operator : Logic  AllPortsSameDT=off  OutDataTypeStr=boolean
  Logical Operator2 : Logic  Operator=NOT  AllPortsSameDT=off  OutDataTypeStr=boolean
  Memory : Memory
  edge : Outport
  wires:
  Logical Operator/1 -> edge/1
  signal/1 -> Memory/1, Logical Operator2/1
  Memory/1 -> Logical Operator/2
  Logical Operator2/1 -> Logical Operator/1

== system Vorlage_Gesamtanlage_v27/Abfüllanlage/Flaschen_data/Flaschengeschwindigkeiten/Anlagenpositionsbestimmung ==
  Flaschenposition : Inport
  Add4 : Sum  Inputs=++++++++++
  Compare To Constant2 : simulink/Logic and Bit Operations/Compare To Constant  relop=>=  const=201  OutDataTypeStr=uint8  ZeroCross=off
  Compare To Constant3 : simulink/Logic and Bit Operations/Compare To Constant  relop=>=  const=205  OutDataTypeStr=uint8  ZeroCross=off
  Compare To Constant4 : simulink/Logic and Bit Operations/Compare To Constant  relop=>=  const=305  OutDataTypeStr=uint8  ZeroCross=off
  Compare To Constant5 : simulink/Logic and Bit Operations/Compare To Constant  relop=>=  const=405  OutDataTypeStr=uint8  ZeroCross=off
  Compare To Constant6 : simulink/Logic and Bit Operations/Compare To Constant  relop=>=  const=504.9  OutDataTypeStr=uint8  ZeroCross=off
  Compare To Constant7 : simulink/Logic and Bit Operations/Compare To Constant  relop=>=  const=604.4  OutDataTypeStr=uint8  ZeroCross=off
  Compare To Constant8 : simulink/Logic and Bit Operations/Compare To Constant  relop=>=  const=610  OutDataTypeStr=uint8  ZeroCross=off
  CompareTo Constant : simulink/Logic and Bit Operations/Compare To Constant  relop=>  const=0  OutDataTypeStr=uint8  ZeroCross=off
  CompareTo Constant1 : simulink/Logic and Bit Operations/Compare To Constant  relop=>=  const=101  OutDataTypeStr=uint8  ZeroCross=off
  Constant9 : Constant
  Anlagenposition : Outport
  wires:
  Constant9/1 -> Add4/1
  CompareTo Constant/1 -> Add4/2
  CompareTo Constant1/1 -> Add4/3
  Compare To Constant2/1 -> Add4/4
  Compare To Constant3/1 -> Add4/5
  Compare To Constant4/1 -> Add4/6
  Compare To Constant5/1 -> Add4/7
  Compare To Constant6/1 -> Add4/8
  Compare To Constant7/1 -> Add4/9
  Compare To Constant8/1 -> Add4/10
  Flaschenposition/1 -> Compare To Constant3/1, Compare To Constant2/1, CompareTo Constant1/1, CompareTo Constant/1, Compare To Constant4/1, Compare To Constant5/1, Compare To Constant6/1, Compare To Constant7/1, Compare To Constant8/1
  Add4/1 -> Anlagenposition/1

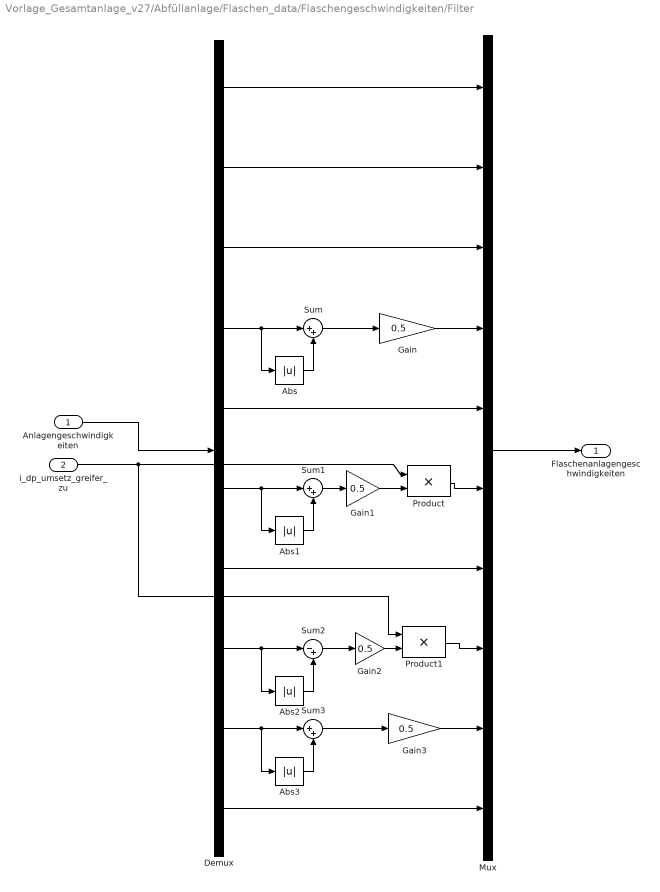
== system Vorlage_Gesamtanlage_v27/Abfüllanlage/Flaschen_data/Flaschengeschwindigkeiten/Filter ==
  Anlagengeschwindigkeiten : Inport
  i_dp_umsetz_greifer_zu : Inport  Port=2
  Abs{,1..3} (4 alike) : Abs  SaturateOnIntegerOverflow=on
  Demux : Demux  Outputs=10
      settings: DisplayOption=none
  Gain{,1..3} (4 alike) : Gain  Gain=0.5  SaturateOnIntegerOverflow=on  OutDataTypeStr=Inherit: Same as input  ParamDataTypeStr=Inherit: Same as input
  Mux : Mux  Inputs=10
  Product : Product  OutDataTypeStr=double  SaturateOnIntegerOverflow=on
  Product1 : Product  OutDataTypeStr=double  SaturateOnIntegerOverflow=on
  Sum : Sum  Inputs=|++  SaturateOnIntegerOverflow=on
  Sum1 : Sum  Inputs=|++  SaturateOnIntegerOverflow=on
  Sum2 : Sum  Inputs=|-+  SaturateOnIntegerOverflow=on
  Sum3 : Sum  Inputs=|++  SaturateOnIntegerOverflow=on
  Flaschenanlagengeschwindigkeiten : Outport
  wires:
  Anlagengeschwindigkeiten/1 -> Demux/1
  Demux/1 -> Mux/1
  Mux/1 -> Flaschenanlagengeschwindigkeiten/1
  Demux/2 -> Mux/2
  Abs/1 -> Sum/2
  Sum/1 -> Gain/1
  Abs1/1 -> Sum1/2
  Gain1/1 -> Product/2
  i_dp_umsetz_greifer_zu/1 -> Product1/1, Product/1
  Abs2/1 -> Sum2/2
  Sum2/1 -> Gain2/1
  Gain2/1 -> Product1/2
  Abs3/1 -> Sum3/2
  Sum3/1 -> Gain3/1
  Demux/10 -> Mux/10
  Sum1/1 -> Gain1/1
  Demux/9 -> Sum3/1, Abs3/1
  Gain3/1 -> Mux/9
  Demux/8 -> Sum2/1, Abs2/1
  Product1/1 -> Mux/8
  Demux/7 -> Mux/7
  Demux/6 -> Sum1/1, Abs1/1
  Product/1 -> Mux/6
  Demux/5 -> Mux/5
  Demux/4 -> Sum/1, Abs/1
  Gain/1 -> Mux/4
  Demux/3 -> Mux/3

== system Vorlage_Gesamtanlage_v27/Abfüllanlage/Flaschen_data/Flaschengeschwindigkeiten/Flaschenabstandsüberwachung ==
  Flaschenpostionen : Inport
  umsetz_pos : Inport  Port=2
  Assignment : Assignment  IndexOptions=Index vector (dialog)  Indices=1  OutputSizes=[1]
  Compare To Constant : simulink/Logic and Bit Operations/Compare To Constant  relop=>=  const=10  OutDataTypeStr=boolean  ZeroCross=off
  Constant1 : Constant  OutDataTypeStr=boolean
  Logical Operator2 : Logic  AllPortsSameDT=off  OutDataTypeStr=boolean
  MATLAB Fcn : MATLABFcn  MATLABFcn=circshift(u, 1)
  Subtract : Sum  Inputs=+-
  Umsetzer darf mitnehmen : Subsystem  TreatAsAtomicUnit=on
  Bewegung möglich : Outport
  wires:
  MATLAB Fcn/1 -> Subtract/1
  Subtract/1 -> Compare To Constant/1
  Flaschenpostionen/1 -> MATLAB Fcn/1, Subtract/2, Umsetzer darf mitnehmen/1(Flaschenpositionen)
  Logical Operator2/1 -> Bewegung möglich/1
  Umsetzer darf mitnehmen/1(darf) -> Logical Operator2/2
  umsetz_pos/1 -> Umsetzer darf mitnehmen/2(umsetzer_pos)
  Assignment/1 -> Logical Operator2/1
  Compare To Constant/1 -> Assignment/1
  Constant1/1 -> Assignment/2

== system Vorlage_Gesamtanlage_v27/Abfüllanlage/Flaschen_data/Flaschenstarter/Flaschenstarter ==
  Flaschenpositionen : Inport
  Flaschenanzahl : Inport  Port=2
  Rising_edge von Flasche : Inport  Port=3
  Assignment : Assignment  IndexOptions=Index vector (port)  Indices=1  OutputSizes=[1]
  Selector : Selector  InputPortWidth=MaxFlaschen  IndexOptions=Index vector (port)  Indices=[1 3]  OutputSizes=1
  Sum : Sum  Inputs=|++  OutDataTypeStr=double  RndMeth=Zero
  Flaschenpositionen mit Starter : Outport
  wires:
  Selector/1 -> Sum/1
  Sum/1 -> Assignment/2
  Flaschenanzahl/1 -> Selector/2, Assignment/3
  Flaschenpositionen/1 -> Assignment/1, Selector/1
  Assignment/1 -> Flaschenpositionen mit Starter/1
  Rising_edge von Flasche/1 -> Sum/2

== system Vorlage_Gesamtanlage_v27/Abfüllanlage/Flaschen_data/Flaschenstarter/in_Flaschenzähler ==
  Signal : Inport
  Constant : Constant
  Constant1 : Constant  Value=0
  Logical Operator : Logic  AllPortsSameDT=off
  Memory : Memory
  Memory1 : Memory
  Relational Operator : RelationalOperator  Operator===  RndMeth=Nearest
  Relational Operator1 : RelationalOperator  Operator===  RndMeth=Nearest
  Sum : Sum  Inputs=|++  OutDataTypeStr=uint16  SaturateOnIntegerOverflow=on
  Rising Edge : Outport
  Count : Outport  Port=2
  wires:
  Signal/1 -> Memory/1, Relational Operator/2
  Constant/1 -> Relational Operator/1
  Relational Operator/1 -> Logical Operator/1
  Constant1/1 -> Relational Operator1/2
  Memory/1 -> Relational Operator1/1
  Relational Operator1/1 -> Logical Operator/2
  Logical Operator/1 -> Sum/1, Rising Edge/1
  Memory1/1 -> Sum/2
  Sum/1 -> Count/1, Memory1/1
